simulink model "balance_robot_real"  (R2024a)
settings: Solver=VariableStepAuto  StartTime=0.0  StopTime=10  RelTol=1e-3
values from neighbouring files (symbols this model uses):
  K_fit = [-0.868061260412 -2.35516956452 -0.346925192861 -4.25165789442 -3.77441240152 -0.248406447853 -3.00338850055 0.151095810733 -21.3173228209 -4.10092881007 -0.868061260412 -2.35516956452 ... (240 elements, 40x6)]    [lqr_fitting_results.mat]
  X = [x1, x2, x1.^2, x2.^2, x1.*x2]    [Calc_K_and_fit.m]    (also in k_calc_chuan_real2.m = [x1, x2, x1sq, x2sq, x1x2])
undefined symbols (not defined in the file or in its folder): Y, Z
libraries: sm_lib x114, nesl_utility x19, slpidlib x3, simulink x1
(part 1 of 3)
settings Model: Creator=zhuho  LastModifiedBy=zhuho

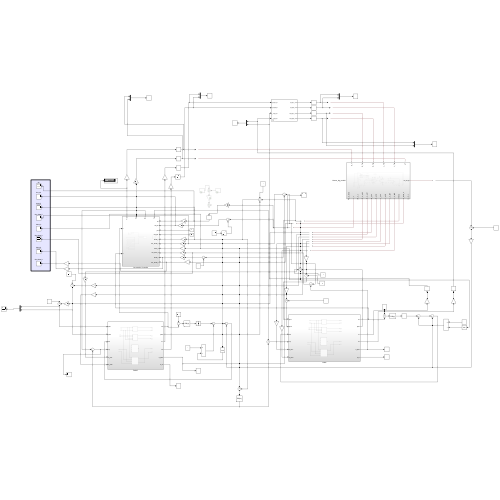
[thumbnail: Simulink's stored preview of the top-level diagram]
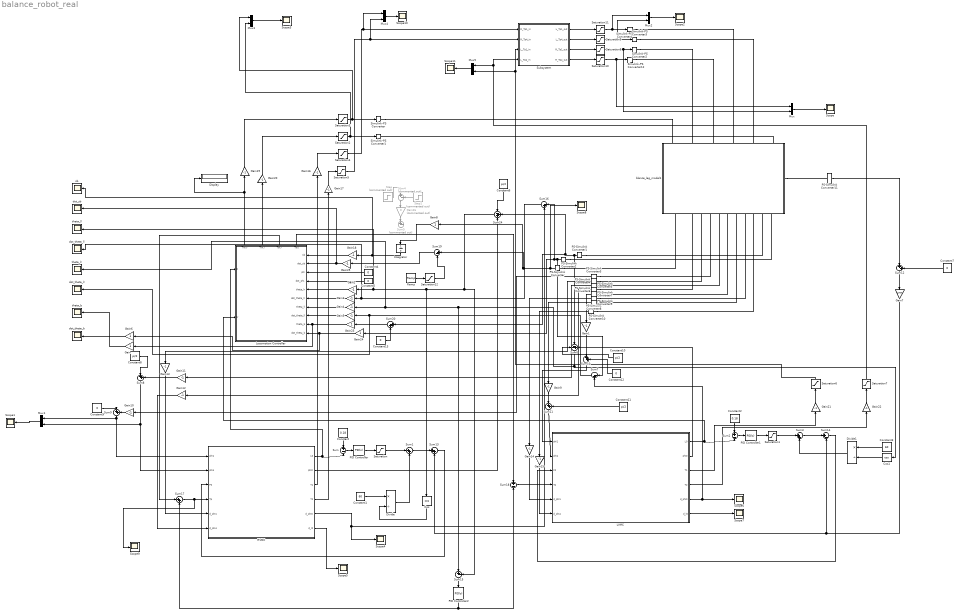
== system balance_robot_real ==
  Constant : Constant  Value=0.18
  Constant1 : Constant  Value=60
  Constant{6,8,10..11} (4 alike) : Constant  Value=pi/2
  Constant{4..5,7,9,12..13} (6 alike) : Constant  Value=0
  Constant2 : Constant  Value=0.18
  Constant3 : Constant  Value=60
  Cos : Trigonometry  Operator=cos
  Cos1 : Trigonometry  Operator=cos
  Display : Display
  Divide : Product  Inputs=*/
  Divide1 : Product  Inputs=*/
  Gain{,6,8,23..24} (5 alike) : Gain
  Gain{1..5,9..22,25} (20 alike) : Gain  Gain=-1
  Gain26 : Gain  Commented=on  Gain=0
  Gain7 : Gain  Gain=1500
  Integrator : Integrator
  LVMC : Subsystem
  Locomotion Controller : Subsystem
      settings: PortSchema="{\"entries\":[{\"content\":{\"sides\":[{\"content\":{\"connectorIds\":[\"In1\",\"In2\"]},\"type\":\"ConnectorPlacement.EquallySpacedRectSide\",\"uuid\":\"9f335f1a-920c-489c-ab23-b2605db4f7eb\"},{\"content\":{\"connectorIds\":[\"In3\",\"In4\",\"In5\",\"In6\",\"In7\",\"In8\",\"In9\",\"In10\",\"In11\",\"In12\"],\"side\":\"RIGHT\"},\"type\":\"ConnectorPlacement.EquallySpacedRectSide\",\"uuid\":\"244eb674-a427-495d-a4b5-69ad08e1900d\"},{\"content\":{\"connectorIds\":[\"Out1\",\"Out2\",\"Out3\",\"Out4\"],\"side\":\"TOP\"},\"type\":\"ConnectorPlacement.EquallySpacedRectSide\",\"uuid\":\"a2322f66-0ec6-4fc3-82d4-b6858da1a4af\"}]},\"type\":\"ConnectorPlacement.EquallySpacedConnector\",\"uuid\":\"7ddcb355-7f50-43e9-8496-f4eccb1abc77\"}],\"packageUris\":[\"http://schema.mathworks.com/mf0/Connector/R2020b\"],\"version\":\"1.0\"}"
  Mux{,1..5} (6 alike) : Mux  Inputs=2
  PID Controller : slpidlib/PID Controller  Controller=PID  Form=Parallel  TimeDomain=Continuous-time  UseExternalTs=off  SampleTime=-1  IntegratorMethod=Forward Euler  FilterMethod=Forward Euler  ControllerParametersSource=internal  P=300  I=0  UseKiTs=off  D=200  UseExternalDerivativeSource=off  N=100  UseFilter=on  TunerSelectOption=Transfer Function Based (PID Tuner App)  InitialConditionSource=internal  InitialConditionForIntegrator=0  InitialConditionForFilter=0  DifferentiatorICPrevScaledInput=0  ExternalReset=none  TrackingMode=off  Kt=1  LimitOutput=off  SatLimitsSource=internal  UpperSaturationLimit=inf  LowerSaturationLimit=-inf  LinearizeAsGain=on  AntiWindupMode=none  Kb=1  LimitIntegrator=off  UpperIntegratorSaturationLimit=inf  LowerIntegratorSaturationLimit=-inf  POutMin=[]  POutMax=[]  IOutMin=[]  IOutMax=[]  DOutMin=[]  DOutMax=[]  NOutMin=[]  NOutMax=[]  SumOutMin=[]  SumOutMax=[]  SaturationOutMin=[]  SaturationOutMax=[]  PParamMin=[]  PParamMax=[]  IParamMin=[]  IParamMax=[]  DParamMin=[]  DParamMax=[]  NParamMin=[]  NParamMax=[]  KbParamMin=[]  KbParamMax=[]  KtParamMin=[]  KtParamMax=[]  KbOutMin=[]  KbOutMax=[]  KtOutMin=[]  KtOutMax=[]  IntegratorOutMin=[]  IntegratorOutMax=[]  FilterOutMin=[]  FilterOutMax=[]  SumI1OutMin=[]  SumI1OutMax=[]  SumI2OutMin=[]  SumI2OutMax=[]  SumI3OutMin=[]  SumI3OutMax=[]  SumI4OutMin=[]  SumI4OutMax=[]  SumDOutMin=[]  SumDOutMax=[]  DifferentiatorOutMin=[]  DifferentiatorOutMax=[]  FilterDiffOutCoefMin=[]  FilterDiffOutCoefMax=[]  ReciprocalOutMin=[]  ReciprocalOutMax=[]  SumDenOutMin=[]  SumDenOutMax=[]  SumNumOutMin=[]  SumNumOutMax=[]  DivideOutMin=[]  DivideOutMax=[]  UdiffTsProdOutMin=[]  UdiffTsProdOutMax=[]  NTsProdOutMin=[]  NTsProdOutMax=[]  UintegralTsProdOutMin=[]  UintegralTsProdOutMax=[]  UngainTsProdOutMin=[]  UngainTsProdOutMax=[]  ClampingZeroOutDataTypeStr=Inherit: Inherit via back propagation  ClampingZeroOutMin=[]  ClampingZeroOutMax=[]  FilterDenConstantOutDataTypeStr=Inherit: Inherit via back propagation  FilterDenConstantOutMin=[]  FilterDenConstantOutMax=[]  PCopyOutDataTypeStr=Inherit: Inherit via back propagation  PCopyOutMin=[]  PCopyOutMax=[]  NCopyOutDataTypeStr=Inherit: Inherit via back propagation  NCopyOutMin=[]  NCopyOutMax=[]  IntegratorContinuousStateAttributes=''  IntegratorStateMustResolveToSignalObject=off  IntegratorRTWStateStorageClass=Auto  FilterContinuousStateAttributes=''  FilterStateMustResolveToSignalObject=off  FilterRTWStateStorageClass=Auto  ParallelPVariant=InternalParameters  IdealPVariant=Disabled  IVariant=InternalParameters  DVariant=InternalParameters  IntegratorVariant=Continuous  SatVariant=Disabled  AWVariant=Passthrough  PCopyVariant=Disabled  TRVariant=Disabled  FdbkBlocksVariant=Forward  IdealPFdbkVariant=Disabled  SatFdbkVariant=Disabled  DerivativeFilterVariant=ContFilter  NVariant=InternalParameters  NCopyVariant=Disabled  FilterICVariant=InternalICsFilter  IntegratorICVariant=InternalICs  ExternalResetVariant=Disabled  TRSumVariant=Passthrough  SumFdbkVariant=Disabled  SumVariant=Sum_PID  TsampFilterVariant=InternalTs  TsampNgainVariant=Passthrough  TsampIntegralVariant=Disabled_SignalSpec  ExternalSaturationOutDataTypeStr=Inherit: Same as second input  DerivativeSourceVariant=ErrorSignal
  PID Controller1 : slpidlib/PID Controller  Controller=PID  Form=Parallel  TimeDomain=Continuous-time  UseExternalTs=off  SampleTime=-1  IntegratorMethod=Forward Euler  FilterMethod=Forward Euler  ControllerParametersSource=internal  P=300  I=0  UseKiTs=off  D=200  UseExternalDerivativeSource=off  N=100  UseFilter=on  TunerSelectOption=Transfer Function Based (PID Tuner App)  InitialConditionSource=internal  InitialConditionForIntegrator=0  InitialConditionForFilter=0  DifferentiatorICPrevScaledInput=0  ExternalReset=none  TrackingMode=off  Kt=1  LimitOutput=off  SatLimitsSource=internal  UpperSaturationLimit=inf  LowerSaturationLimit=-inf  LinearizeAsGain=on  AntiWindupMode=none  Kb=1  LimitIntegrator=off  UpperIntegratorSaturationLimit=inf  LowerIntegratorSaturationLimit=-inf  POutMin=[]  POutMax=[]  IOutMin=[]  IOutMax=[]  DOutMin=[]  DOutMax=[]  NOutMin=[]  NOutMax=[]  SumOutMin=[]  SumOutMax=[]  SaturationOutMin=[]  SaturationOutMax=[]  PParamMin=[]  PParamMax=[]  IParamMin=[]  IParamMax=[]  DParamMin=[]  DParamMax=[]  NParamMin=[]  NParamMax=[]  KbParamMin=[]  KbParamMax=[]  KtParamMin=[]  KtParamMax=[]  KbOutMin=[]  KbOutMax=[]  KtOutMin=[]  KtOutMax=[]  IntegratorOutMin=[]  IntegratorOutMax=[]  FilterOutMin=[]  FilterOutMax=[]  SumI1OutMin=[]  SumI1OutMax=[]  SumI2OutMin=[]  SumI2OutMax=[]  SumI3OutMin=[]  SumI3OutMax=[]  SumI4OutMin=[]  SumI4OutMax=[]  SumDOutMin=[]  SumDOutMax=[]  DifferentiatorOutMin=[]  DifferentiatorOutMax=[]  FilterDiffOutCoefMin=[]  FilterDiffOutCoefMax=[]  ReciprocalOutMin=[]  ReciprocalOutMax=[]  SumDenOutMin=[]  SumDenOutMax=[]  SumNumOutMin=[]  SumNumOutMax=[]  DivideOutMin=[]  DivideOutMax=[]  UdiffTsProdOutMin=[]  UdiffTsProdOutMax=[]  NTsProdOutMin=[]  NTsProdOutMax=[]  UintegralTsProdOutMin=[]  UintegralTsProdOutMax=[]  UngainTsProdOutMin=[]  UngainTsProdOutMax=[]  ClampingZeroOutDataTypeStr=Inherit: Inherit via back propagation  ClampingZeroOutMin=[]  ClampingZeroOutMax=[]  FilterDenConstantOutDataTypeStr=Inherit: Inherit via back propagation  FilterDenConstantOutMin=[]  FilterDenConstantOutMax=[]  PCopyOutDataTypeStr=Inherit: Inherit via back propagation  PCopyOutMin=[]  PCopyOutMax=[]  NCopyOutDataTypeStr=Inherit: Inherit via back propagation  NCopyOutMin=[]  NCopyOutMax=[]  IntegratorContinuousStateAttributes=''  IntegratorStateMustResolveToSignalObject=off  IntegratorRTWStateStorageClass=Auto  FilterContinuousStateAttributes=''  FilterStateMustResolveToSignalObject=off  FilterRTWStateStorageClass=Auto  ParallelPVariant=InternalParameters  IdealPVariant=Disabled  IVariant=InternalParameters  DVariant=InternalParameters  IntegratorVariant=Continuous  SatVariant=Disabled  AWVariant=Passthrough  PCopyVariant=Disabled  TRVariant=Disabled  FdbkBlocksVariant=Forward  IdealPFdbkVariant=Disabled  SatFdbkVariant=Disabled  DerivativeFilterVariant=ContFilter  NVariant=InternalParameters  NCopyVariant=Disabled  FilterICVariant=InternalICsFilter  IntegratorICVariant=InternalICs  ExternalResetVariant=Disabled  TRSumVariant=Passthrough  SumFdbkVariant=Disabled  SumVariant=Sum_PID  TsampFilterVariant=InternalTs  TsampNgainVariant=Passthrough  TsampIntegralVariant=Disabled_SignalSpec  ExternalSaturationOutDataTypeStr=Inherit: Same as second input  DerivativeSourceVariant=ErrorSignal
  PID Controller2 : slpidlib/PID Controller  Controller=PID  Form=Parallel  TimeDomain=Continuous-time  UseExternalTs=off  SampleTime=-1  IntegratorMethod=Forward Euler  FilterMethod=Forward Euler  ControllerParametersSource=internal  P=500  I=0  UseKiTs=off  D=100  UseExternalDerivativeSource=off  N=100  UseFilter=on  TunerSelectOption=Transfer Function Based (PID Tuner App)  InitialConditionSource=internal  InitialConditionForIntegrator=0  InitialConditionForFilter=0  DifferentiatorICPrevScaledInput=0  ExternalReset=none  TrackingMode=off  Kt=1  LimitOutput=off  SatLimitsSource=internal  UpperSaturationLimit=inf  LowerSaturationLimit=-inf  LinearizeAsGain=on  AntiWindupMode=none  Kb=1  LimitIntegrator=off  UpperIntegratorSaturationLimit=inf  LowerIntegratorSaturationLimit=-inf  POutMin=[]  POutMax=[]  IOutMin=[]  IOutMax=[]  DOutMin=[]  DOutMax=[]  NOutMin=[]  NOutMax=[]  SumOutMin=[]  SumOutMax=[]  SaturationOutMin=[]  SaturationOutMax=[]  PParamMin=[]  PParamMax=[]  IParamMin=[]  IParamMax=[]  DParamMin=[]  DParamMax=[]  NParamMin=[]  NParamMax=[]  KbParamMin=[]  KbParamMax=[]  KtParamMin=[]  KtParamMax=[]  KbOutMin=[]  KbOutMax=[]  KtOutMin=[]  KtOutMax=[]  IntegratorOutMin=[]  IntegratorOutMax=[]  FilterOutMin=[]  FilterOutMax=[]  SumI1OutMin=[]  SumI1OutMax=[]  SumI2OutMin=[]  SumI2OutMax=[]  SumI3OutMin=[]  SumI3OutMax=[]  SumI4OutMin=[]  SumI4OutMax=[]  SumDOutMin=[]  SumDOutMax=[]  DifferentiatorOutMin=[]  DifferentiatorOutMax=[]  FilterDiffOutCoefMin=[]  FilterDiffOutCoefMax=[]  ReciprocalOutMin=[]  ReciprocalOutMax=[]  SumDenOutMin=[]  SumDenOutMax=[]  SumNumOutMin=[]  SumNumOutMax=[]  DivideOutMin=[]  DivideOutMax=[]  UdiffTsProdOutMin=[]  UdiffTsProdOutMax=[]  NTsProdOutMin=[]  NTsProdOutMax=[]  UintegralTsProdOutMin=[]  UintegralTsProdOutMax=[]  UngainTsProdOutMin=[]  UngainTsProdOutMax=[]  ClampingZeroOutDataTypeStr=Inherit: Inherit via back propagation  ClampingZeroOutMin=[]  ClampingZeroOutMax=[]  FilterDenConstantOutDataTypeStr=Inherit: Inherit via back propagation  FilterDenConstantOutMin=[]  FilterDenConstantOutMax=[]  PCopyOutDataTypeStr=Inherit: Inherit via back propagation  PCopyOutMin=[]  PCopyOutMax=[]  NCopyOutDataTypeStr=Inherit: Inherit via back propagation  NCopyOutMin=[]  NCopyOutMax=[]  IntegratorContinuousStateAttributes=''  IntegratorStateMustResolveToSignalObject=off  IntegratorRTWStateStorageClass=Auto  FilterContinuousStateAttributes=''  FilterStateMustResolveToSignalObject=off  FilterRTWStateStorageClass=Auto  ParallelPVariant=InternalParameters  IdealPVariant=Disabled  IVariant=InternalParameters  DVariant=InternalParameters  IntegratorVariant=Continuous  SatVariant=Disabled  AWVariant=Passthrough  PCopyVariant=Disabled  TRVariant=Disabled  FdbkBlocksVariant=Forward  IdealPFdbkVariant=Disabled  SatFdbkVariant=Disabled  DerivativeFilterVariant=ContFilter  NVariant=InternalParameters  NCopyVariant=Disabled  FilterICVariant=InternalICsFilter  IntegratorICVariant=InternalICs  ExternalResetVariant=Disabled  TRSumVariant=Passthrough  SumFdbkVariant=Disabled  SumVariant=Sum_PID  TsampFilterVariant=InternalTs  TsampNgainVariant=Passthrough  TsampIntegralVariant=Disabled_SignalSpec  ExternalSaturationOutDataTypeStr=Inherit: Same as second input  DerivativeSourceVariant=ErrorSignal
  PS-Simulink Converter{,1..11} (12 alike) : nesl_utility/PS-Simulink Converter  PhysicalDomain=network_engine_domain  SubClassName=ps_output  LeftPortType=input  RightPortType=output  PseudoPeriodic=off  Frequencies=[]  VectorFormat=inherit  Unit=inherit  AffineConversion=off
  RVMC : Subsystem
  Ramp : simulink/Sources/Ramp  slope=2  start=0.2  InitialOutput=0
  Saturation : Saturate  UpperLimit=9  LowerLimit=-9
  Saturation1 : Saturate  UpperLimit=9  LowerLimit=-9
  Saturation{8..11} (4 alike) : Saturate  UpperLimit=100  LowerLimit=-100
  Saturation12 : Saturate  UpperLimit=0  LowerLimit=0
  Saturation2 : Saturate  UpperLimit=2.7  LowerLimit=-2.7
  Saturation3 : Saturate  UpperLimit=2.7  LowerLimit=-2.7
  Saturation{4..7} (4 alike) : Saturate  UpperLimit=20  LowerLimit=-20
  Scope{,1..11} (12 alike) : Scope
  Simulink-PS Converter{,1..4,12} (6 alike) : nesl_utility/Simulink-PS Converter  PhysicalDomain=network_engine_domain  SubClassName=ps_input  LeftPortType=input  RightPortType=output  PseudoPeriodic=off  Frequencies=[]  NoiseDistribution=none  NoiseParameters=[]  Unit=1  AffineConversion=off  FilteringAndDerivatives=provide  SimscapeFilterOrder=1  InputFilterTimeConstant=0.001  UdotUserProvided=0
  Step : Step  Commented=on  Time=0.8  After=3  SampleTime=0
  Step1 : Step  Commented=on  Time=5  After=3  SampleTime=0
  Subsystem : Subsystem  mask{Jump_time=0, Jump_torque=0}
      mask DialogControl ParameterGroupVar Prompt: 参数
  Sum : Sum  Inputs=+|-
  Sum{1,3,8..13,17,20} (10 alike) : Sum  Inputs=|++
  Sum14 : Sum  Inputs=|+-
  Sum15 : Sum  Inputs=|+-
  Sum16 : Sum  Inputs=|-+
  Sum18 : Sum  Inputs=+|-
  Sum19 : Sum  Inputs=|+-
  Sum2 : Sum  Inputs=+|-
  Sum24 : Sum  Inputs=--+
  Sum4 : Sum  Commented=on  Inputs=|+-
  Sum5 : Sum  Commented=on  Inputs=|+-
  Sum6 : Sum  Inputs=--+
  Sum7 : Sum  Inputs=|-+
  blance_leg_model1 : Subsystem
      settings: PortSchema="{\"entries\":[{\"content\":{\"sides\":[{\"content\":{\"connectorIds\":[\"LConn1\",\"LConn2\",\"LConn3\",\"LConn4\",\"LConn5\",\"LConn6\"]},\"type\":\"ConnectorPlacement.EquallySpacedRectSide\",\"uuid\":\"04fe8e60-572e-417f-9580-631ec97f8421\"},{\"content\":{\"connectorIds\":[\"RConn1\",\"RConn2\",\"RConn3\",\"RConn4\",\"RConn5\",\"RConn6\",\"RConn7\",\"RConn8\",\"RConn9\",\"RConn10\",\"RConn11\",\"RConn12\",\"RConn13\",\"RConn14\"],\"side\":\"RIGHT\"},\"type\":\"ConnectorPlacement.EquallySpacedRectSide\",\"uuid\":\"8cd76564-77eb-4f45-a98d-9ceca116fdaa\"},{\"content\":{\"side\":\"TOP\"},\"type\":\"ConnectorPlacement.EquallySpacedRectSide\",\"uuid\":\"cf774899-dead-43c6-9d06-3eadf5f34dd8\"},{\"content\":{\"connectorIds\":[\"RConn15\"],\"side\":\"BOTTOM\"},\"type\":\"ConnectorPlacement.EquallySpacedRectSide\",\"uuid\":\"6b0f740d-a430-486c-abbf-1036029346ea\"}]},\"type\":\"ConnectorPlacement.EquallySpacedConnector\",\"uuid\":\"5fab14ca-8df0-4e19-8db5-40800b78baae\"}],\"packageUris\":[\"http://schema.mathworks.com/mf0/Connector/R2020b\"],\"version\":\"1.0\"}"
  dot_sb : Scope
  dot_theta_b : Scope
  dot_theta_ll : Scope
  dot_theta_lr : Scope
  sb : Scope
  theta_b : Scope
  theta_ll : Scope
  theta_lr : Scope
  wires:
  Gain24/1 -> Gain6/1, Locomotion Controller/12(dot_theta_b)
  RVMC/6(d_l0) -> Scope5/1
  Gain6/1 -> dot_theta_b/1
  Sum19/1 -> Gain25/1
  Ramp/1 -> Saturation12/1
  LVMC/6(d_l0) -> Scope7/1
  Sum16/1 -> dot_theta_ll/1, Gain3/1
  Mux2/1 -> Scope2/1
  Mux3/1 -> Scope3/1
  Sum10/1 -> LVMC/1(phi1)
  Saturation2/1 -> Mux3/2, Simulink-PS Converter1/1
  RVMC/5(d_phi0) -> Scope4/1, Sum16/2
  Saturation7/1 -> Mux5/1, Subsystem/4(L_Tp4_in)
  Saturation4/1 -> Mux4/1, Subsystem/1(R_Tp1_in)
  Gain26/1 -> Sum5/1
  Sum15/1 -> PID Controller2/1
  Constant12/1 -> Sum10/2
  Gain14/1 -> LVMC/5(d_phi1)
  LVMC/2(phi0) -> Sum6/3
  Subsystem/4(R_Tp4_out) -> Saturation10/1
  Subsystem/1(L_Tp1_out) -> Saturation11/1
  Sum6/1 -> Cos1/1, theta_lr/1, Gain4/1, Sum15/1
  Divide1/1 -> Sum3/2
  Gain10/1 -> Sum9/2
  Gain9/1 -> Sum11/1
  Sum4/1 -> Gain26/1
  Step1/1 -> Sum4/2
  Mux/1 -> Scope/1
  Locomotion Controller/1(Tlw,r) -> Display/1, Gain19/1
  Constant4/1 -> Locomotion Controller/5(phi)
  Locomotion Controller/3(Tbl,r) -> Sum17/1
  PS-Simulink Converter11/1 -> Sum12/1
  Sum1/1 -> Sum13/1
  Subsystem/3(R_Tp1_out) -> Saturation8/1
  Saturation8/1 -> Mux/2, Simulink-PS Converter2/1
  Gain1/1 -> Sum10/1
  Gain20/1 -> Saturation2/1
  PS-Simulink Converter6/1 -> Gain12/1
  Mux1/1 -> Scope1/1
  Gain23/1 -> Gain/1, Locomotion Controller/11(theta_b)
  Gain17/1 -> Saturation5/1
  Gain16/1 -> Saturation4/1
  Gain19/1 -> Saturation3/1
  Cos1/1 -> Divide1/2
  LVMC/4(T2) -> Gain22/1
  Constant/1 -> Sum/1
  LVMC/3(T1) -> Gain21/1
  Sum3/1 -> Sum14/1
  Gain18/1 -> Locomotion Controller/3(sb)
  PS-Simulink Converter/1 -> Sum19/1, Gain8/1, Scope8/1
  PS-Simulink Converter2/1 -> Sum7/1, Gain24/1, Sum16/1
  Gain5/1 -> Locomotion Controller/10(dot_theta_ll)
  Constant10/1 -> Sum6/1
  RVMC/4(T2) -> Gain17/1
  Gain11/1 -> Sum8/2
  Sum9/1 -> RVMC/1(phi1), Mux1/1
  Saturation/1 -> Sum1/1
  Gain13/1 -> RVMC/5(d_phi1)
  Constant6/1 -> Sum24/1
  PID Controller/1 -> Saturation/1
  RVMC/1(L0) -> Sum/2, Locomotion Controller/1(ll)
  PS-Simulink Converter9/1 -> Gain9/1
  PID Controller1/1 -> Saturation1/1
  Gain15/1 -> LVMC/6(d_phi4)
  Constant5/1 -> Locomotion Controller/6(dot_phi.)
  Cos/1 -> Divide/2
  RVMC/3(T1) -> Gain16/1
  Sum7/1 -> dot_theta_lr/1, Gain5/1
  PS-Simulink Converter3/1 -> Gain10/1
  PS-Simulink Converter5/1 -> Gain11/1
  Gain3/1 -> Locomotion Controller/8(dot_theta_lr)
  Constant9/1 -> Sum9/1
  Sum2/1 -> PID Controller1/1
  Saturation1/1 -> Sum3/1
  PS-Simulink Converter10/1 -> Gain15/1
  PS-Simulink Converter8/1 -> Gain14/1
  Constant11/1 -> Sum11/2
  Constant2/1 -> Sum2/1
  Constant8/1 -> Sum8/1
  PS-Simulink Converter7/1 -> Gain1/1
  Gain2/1 -> Locomotion Controller/7(theta_lr)
  Gain21/1 -> Saturation6/1
  Sum12/1 -> Gain7/1
  Integrator/1 -> Gain18/1, sb/1
  Saturation5/1 -> Mux4/2, Subsystem/2(R_Tp4_in)
  Gain25/1 -> dot_sb/1, Locomotion Controller/4(dot_sb)
  Step/1 -> Sum4/1
  Gain22/1 -> Saturation7/1
  PID Controller2/1 -> Sum17/2, Sum18/2
  Subsystem/2(L_Tp4_out) -> Saturation9/1
  Constant7/1 -> Sum12/2
  Sum11/1 -> LVMC/2(phi4)
  Sum24/1 -> Sum15/2, theta_ll/1, Gain2/1, Cos/1
  Gain7/1 -> Sum14/2, Sum13/2
  Sum13/1 -> RVMC/3(F0)
  Gain12/1 -> RVMC/6(d_phi4)
  Sum14/1 -> LVMC/3(F0)
  Saturation12/1 -> Sum19/2
  Gain4/1 -> Locomotion Controller/9(theta_ll)
  Locomotion Controller/2(Tlw,l) -> Gain20/1
  PS-Simulink Converter4/1 -> Gain13/1
  Saturation11/1 -> Mux2/1, Simulink-PS Converter4/1
  LVMC/1(L0) -> Sum2/2, Locomotion Controller/2(lr)
  Sum18/1 -> LVMC/4(Tp)
  Saturation3/1 -> Mux3/1, Simulink-PS Converter/1
  Sum17/1 -> Scope9/1, RVMC/4(Tp)
  Constant1/1 -> Divide/1
  Sum/1 -> PID Controller/1
  Divide/1 -> Sum1/2
  Locomotion Controller/4(Tbl,l) -> Sum18/1
  RVMC/2(phi0) -> Sum24/3
  LVMC/5(d_phi0) -> Sum7/2, Scope6/1
  Saturation10/1 -> Mux/1, Simulink-PS Converter12/1
  Saturation6/1 -> Mux5/2, Subsystem/3(L_Tp1_in)
  Constant3/1 -> Divide1/1
  PS-Simulink Converter1/1 -> Sum20/1, Sum24/2, Sum6/2
  Sum8/1 -> RVMC/2(phi4), Mux1/2
  Saturation9/1 -> Mux2/2, Simulink-PS Converter3/1
  Gain/1 -> theta_b/1
  Gain8/1 -> Integrator/1
  Constant13/1 -> Sum20/2
  Sum20/1 -> Gain23/1
  Mux4/1 -> Scope10/1
  Mux5/1 -> Scope11/1
  connections:
  Simulink-PS Converter2/RConn1 -- blance_leg_model1/LConn2
  PS-Simulink Converter2/LConn1 -- blance_leg_model1/RConn13
  PS-Simulink Converter5/LConn1 -- blance_leg_model1/RConn7
  Simulink-PS Converter/RConn1 -- blance_leg_model1/LConn1
  PS-Simulink Converter8/LConn1 -- blance_leg_model1/RConn10
  PS-Simulink Converter7/LConn1 -- blance_leg_model1/RConn8
  blance_leg_model1/RConn15 -- PS-Simulink Converter11/LConn1
  PS-Simulink Converter10/LConn1 -- blance_leg_model1/RConn11
  Simulink-PS Converter4/RConn1 -- blance_leg_model1/LConn4
  PS-Simulink Converter/LConn1 -- blance_leg_model1/RConn2
  Simulink-PS Converter3/RConn1 -- blance_leg_model1/LConn5
  PS-Simulink Converter4/LConn1 -- blance_leg_model1/RConn5
  Simulink-PS Converter12/RConn1 -- blance_leg_model1/LConn3
  PS-Simulink Converter1/LConn1 -- blance_leg_model1/RConn12
  PS-Simulink Converter6/LConn1 -- blance_leg_model1/RConn4
  blance_leg_model1/LConn6 -- Simulink-PS Converter1/RConn1
  PS-Simulink Converter9/LConn1 -- blance_leg_model1/RConn9
  PS-Simulink Converter3/LConn1 -- blance_leg_model1/RConn6

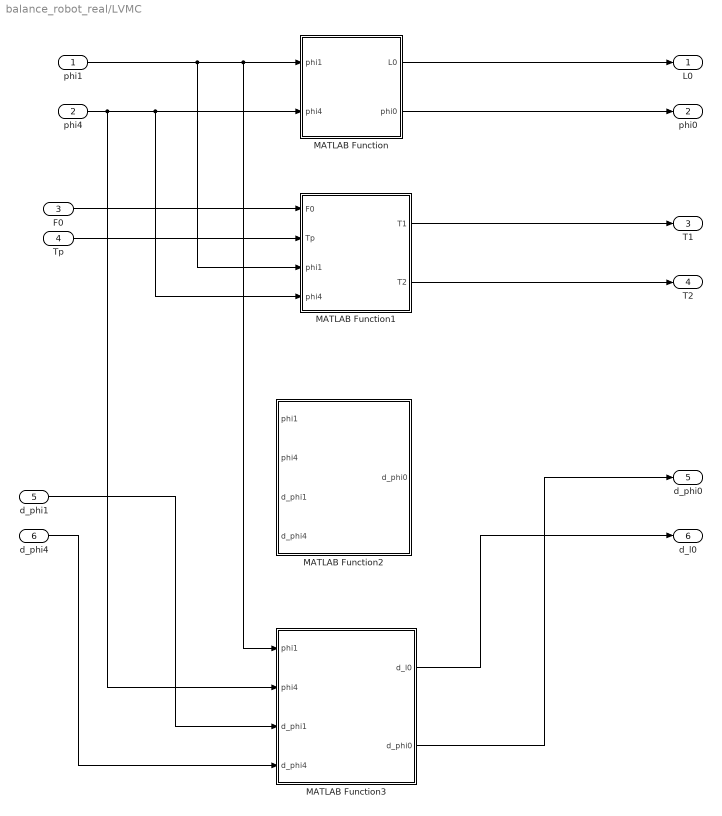
== system balance_robot_real/LVMC ==
  phi1 : Inport
  phi4 : Inport  Port=2
  F0 : Inport  Port=3
  Tp : Inport  Port=4
  d_phi1 : Inport  Port=5
  d_phi4 : Inport  Port=6
  MATLAB Function : MATLAB Function  TreatAsAtomicUnit=on
  MATLAB Function1 : MATLAB Function  TreatAsAtomicUnit=on
  MATLAB Function2 : MATLAB Function  TreatAsAtomicUnit=on
  MATLAB Function3 : MATLAB Function  TreatAsAtomicUnit=on
  L0 : Outport
  phi0 : Outport  Port=2
  T1 : Outport  Port=3
  T2 : Outport  Port=4
  d_phi0 : Outport  Port=5
  d_l0 : Outport  Port=6
  wires:
  phi1/1 -> MATLAB Function1/3(phi1), MATLAB Function3/1(phi1), MATLAB Function/1(phi1)
  phi4/1 -> MATLAB Function3/2(phi4), MATLAB Function1/4(phi4), MATLAB Function/2(phi4)
  F0/1 -> MATLAB Function1/1(F0)
  Tp/1 -> MATLAB Function1/2(Tp)
  MATLAB Function/1(L0) -> L0/1
  MATLAB Function/2(phi0) -> phi0/1
  MATLAB Function1/1(T1) -> T1/1
  MATLAB Function1/2(T2) -> T2/1
  d_phi1/1 -> MATLAB Function3/3(d_phi1)
  d_phi4/1 -> MATLAB Function3/4(d_phi4)
  MATLAB Function3/2(d_phi0) -> d_phi0/1
  MATLAB Function3/1(d_l0) -> d_l0/1

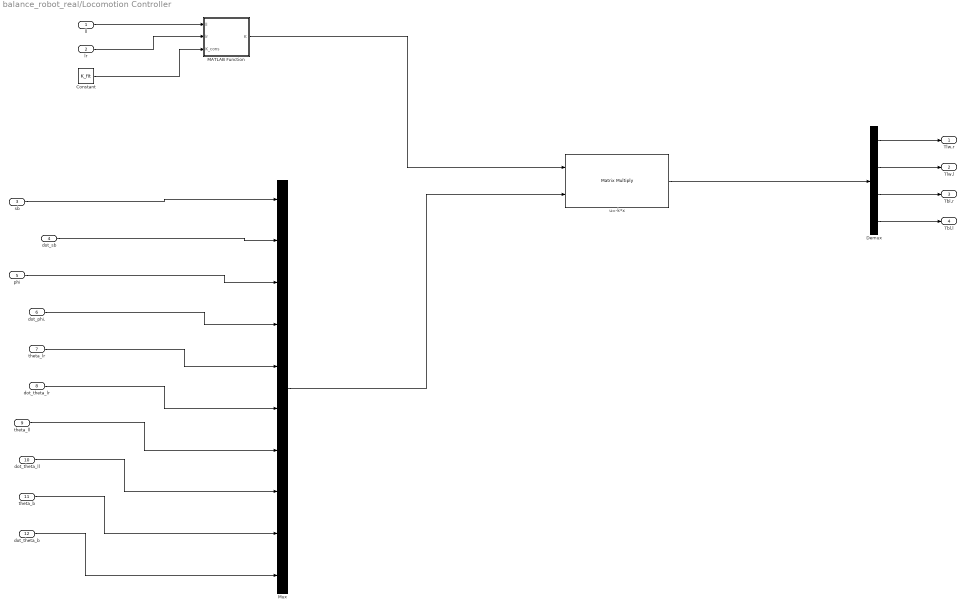
== system balance_robot_real/Locomotion Controller ==
  ll : Inport
  lr : Inport  Port=2
  sb : Inport  Port=3
  dot_sb : Inport  Port=4
  phi : Inport  Port=5
  dot_phi. : Inport  Port=6
  theta_lr : Inport  Port=7
  dot_theta_lr : Inport  Port=8
  theta_ll : Inport  Port=9
  dot_theta_ll : Inport  Port=10
  theta_b : Inport  Port=11
  dot_theta_b : Inport  Port=12
  Constant : Constant  Value=K_fit
  Demux : Demux
  MATLAB Function : MATLAB Function  TreatAsAtomicUnit=on
  Mux : Mux  Inputs=10
  u=-k*x : Product  Multiplication=Matrix(*)
  Tlw,r : Outport
  Tlw,l : Outport  Port=2
  Tbl,r : Outport  Port=3
  Tbl,l : Outport  Port=4
  wires:
  ll/1 -> MATLAB Function/1(ll)
  lr/1 -> MATLAB Function/2(lr)
  Constant/1 -> MATLAB Function/3(K_cons)
  sb/1 -> Mux/1
  dot_sb/1 -> Mux/2
  phi/1 -> Mux/3
  dot_phi./1 -> Mux/4
  theta_lr/1 -> Mux/5
  dot_theta_lr/1 -> Mux/6
  theta_ll/1 -> Mux/7
  dot_theta_ll/1 -> Mux/8
  theta_b/1 -> Mux/9
  dot_theta_b/1 -> Mux/10
  MATLAB Function/1(K) -> u=-k*x/1
  Mux/1 -> u=-k*x/2
  u=-k*x/1 -> Demux/1
  Demux/1 -> Tlw,r/1
  Demux/2 -> Tlw,l/1
  Demux/3 -> Tbl,r/1
  Demux/4 -> Tbl,l/1

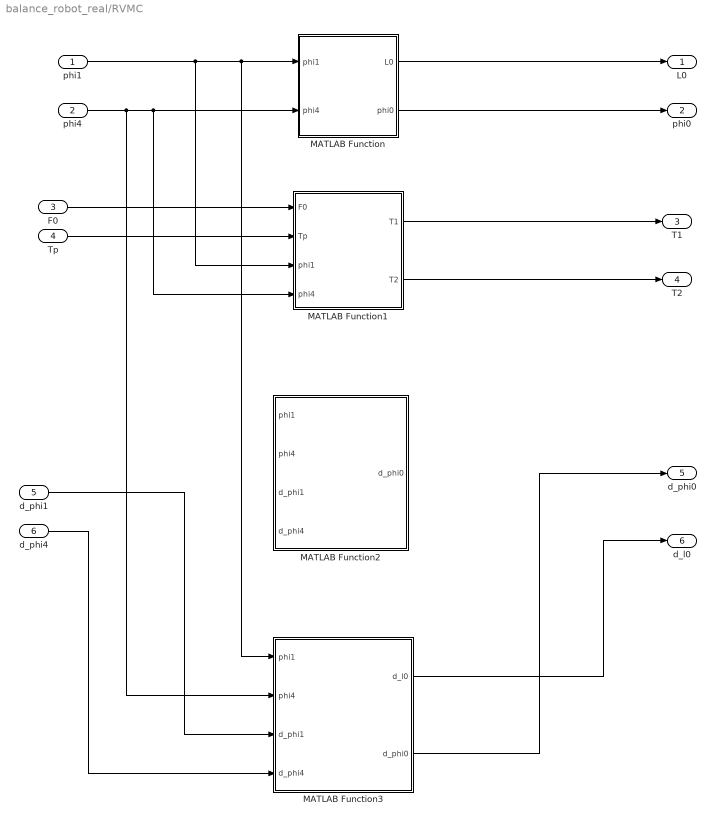
== system balance_robot_real/RVMC ==
  phi1 : Inport
  phi4 : Inport  Port=2
  F0 : Inport  Port=3
  Tp : Inport  Port=4
  d_phi1 : Inport  Port=5
  d_phi4 : Inport  Port=6
  MATLAB Function : MATLAB Function  TreatAsAtomicUnit=on
  MATLAB Function1 : MATLAB Function  TreatAsAtomicUnit=on
  MATLAB Function2 : MATLAB Function  TreatAsAtomicUnit=on
  MATLAB Function3 : MATLAB Function  TreatAsAtomicUnit=on
  L0 : Outport
  phi0 : Outport  Port=2
  T1 : Outport  Port=3
  T2 : Outport  Port=4
  d_phi0 : Outport  Port=5
  d_l0 : Outport  Port=6
  wires:
  phi1/1 -> MATLAB Function1/3(phi1), MATLAB Function3/1(phi1), MATLAB Function/1(phi1)
  phi4/1 -> MATLAB Function3/2(phi4), MATLAB Function1/4(phi4), MATLAB Function/2(phi4)
  F0/1 -> MATLAB Function1/1(F0)
  Tp/1 -> MATLAB Function1/2(Tp)
  MATLAB Function/1(L0) -> L0/1
  MATLAB Function/2(phi0) -> phi0/1
  MATLAB Function1/1(T1) -> T1/1
  MATLAB Function1/2(T2) -> T2/1
  d_phi1/1 -> MATLAB Function3/3(d_phi1)
  d_phi4/1 -> MATLAB Function3/4(d_phi4)
  MATLAB Function3/2(d_phi0) -> d_phi0/1
  MATLAB Function3/1(d_l0) -> d_l0/1

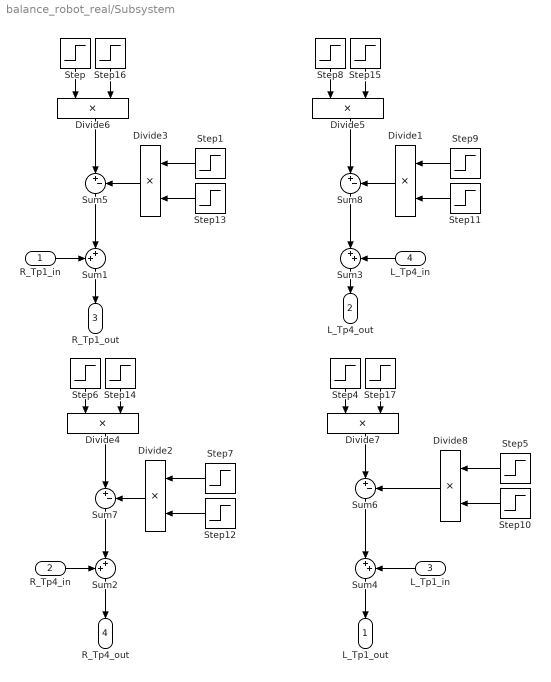
== system balance_robot_real/Subsystem ==
  R_Tp1_in : Inport
  R_Tp4_in : Inport  Port=2
  L_Tp1_in : Inport  Port=3
  L_Tp4_in : Inport  Port=4
  Divide{1..8} (8 alike) : Product  Inputs=**
  Step : Step  Time=Jump_time  After=-Jump_torque  SampleTime=0
  Step1 : Step  Time=Jump_time+0.15  After=-Jump_torque  SampleTime=0
  Step{10..13} (4 alike) : Step  Time=Jump_time+0.4  Before=1  After=0  SampleTime=0
  Step{14..17} (4 alike) : Step  Time=Jump_time+0.2  Before=1  After=0  SampleTime=0
  Step4 : Step  Time=Jump_time  After=-Jump_torque  SampleTime=0
  Step5 : Step  Time=Jump_time+0.15  After=-Jump_torque  SampleTime=0
  Step6 : Step  Time=Jump_time  After=Jump_torque  SampleTime=0
  Step7 : Step  Time=Jump_time+0.15  After=Jump_torque  SampleTime=0
  Step8 : Step  Time=Jump_time  After=Jump_torque  SampleTime=0
  Step9 : Step  Time=Jump_time+0.15  After=Jump_torque  SampleTime=0
  Sum1 : Sum  Inputs=++|
  Sum2 : Sum  Inputs=++|
  Sum3 : Sum  Inputs=|++
  Sum4 : Sum  Inputs=|++
  Sum{5..8} (4 alike) : Sum  Inputs=|+-
  L_Tp1_out : Outport
  L_Tp4_out : Outport  Port=2
  R_Tp1_out : Outport  Port=3
  R_Tp4_out : Outport  Port=4
  wires:
  Step9/1 -> Divide1/1
  Divide6/1 -> Sum5/1
  Step14/1 -> Divide4/2
  Step5/1 -> Divide8/1
  R_Tp1_in/1 -> Sum1/1
  Sum1/1 -> R_Tp1_out/1
  Step4/1 -> Divide7/1
  Divide1/1 -> Sum8/2
  Divide5/1 -> Sum8/1
  Step/1 -> Divide6/1
  Step17/1 -> Divide7/2
  Step6/1 -> Divide4/1
  Sum3/1 -> L_Tp4_out/1
  Step15/1 -> Divide5/2
  Sum2/1 -> R_Tp4_out/1
  Sum4/1 -> L_Tp1_out/1
  R_Tp4_in/1 -> Sum2/1
  Divide7/1 -> Sum6/1
  Sum5/1 -> Sum1/2
  Step10/1 -> Divide8/2
  L_Tp4_in/1 -> Sum3/2
  Step12/1 -> Divide2/2
  Step13/1 -> Divide3/2
  Divide2/1 -> Sum7/2
  Step11/1 -> Divide1/2
  Sum8/1 -> Sum3/1
  Divide8/1 -> Sum6/2
  Step8/1 -> Divide5/1
  Sum7/1 -> Sum2/2
  Divide4/1 -> Sum7/1
  L_Tp1_in/1 -> Sum4/2
  Step7/1 -> Divide2/1
  Step1/1 -> Divide3/1
  Divide3/1 -> Sum5/2
  Sum6/1 -> Sum4/1
  Step16/1 -> Divide6/2
